simulink model "Q4_V2"  (R2021b)
settings: Solver=VariableStepAuto  StartTime=0.0  StopTime=10  MaxStep=0.0001  RelTol=1e-3
undefined symbols (not defined in the file): a0, a1, a2, b, P0, theta_zero, wn, zeta
libraries: cstblocks x2
settings Model: Creator=mahdi  LastModifiedBy=mahdi

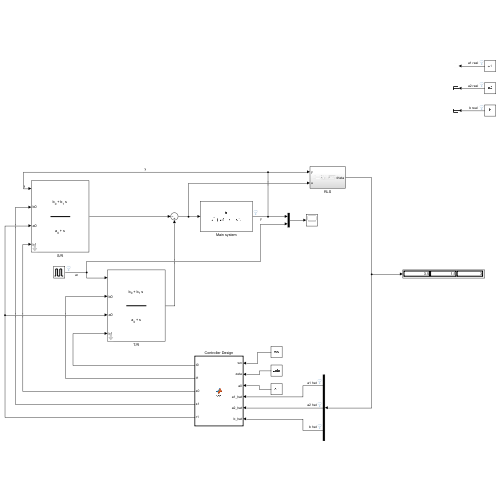
[thumbnail: Simulink's stored preview of the top-level diagram]
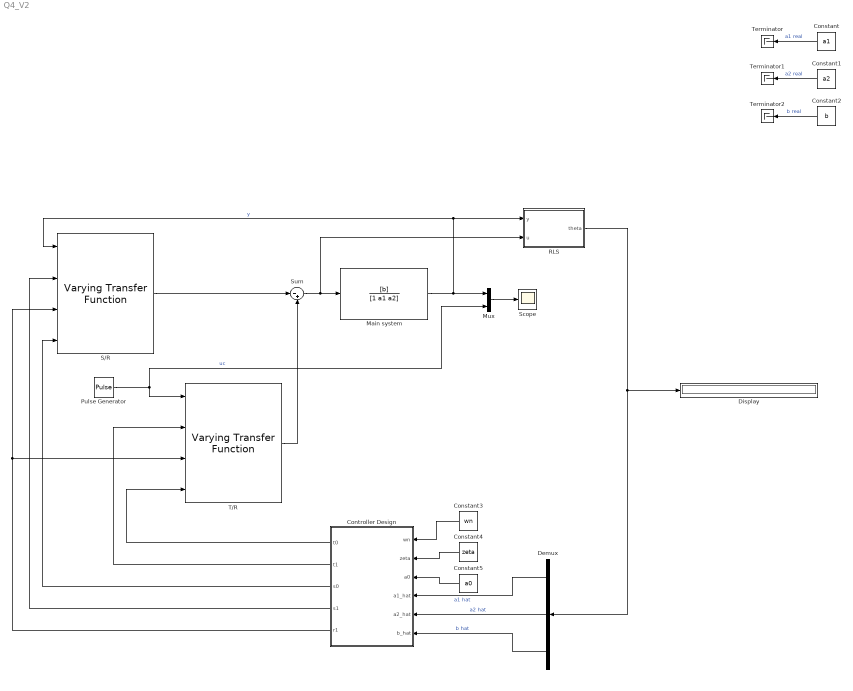
== system Q4_V2 ==
  Constant : Constant  Value=a1
  Constant1 : Constant  Value=a2
  Constant2 : Constant  Value=b
  Constant3 : Constant  Value=wn
  Constant4 : Constant  Value=zeta
  Constant5 : Constant  Value=a0
  Controller Design : MATLAB Function  TreatAsAtomicUnit=on
  Demux : Demux  Outputs=3
  Display : Display
  Main system : TransferFcn  Numerator=[b]  Denominator=[1 a1 a2]
  Mux : Mux  Inputs=2
  Pulse Generator : DiscretePulseGenerator  PulseType=Time based  Period=5  PulseWidth=50
  RLS : Subsystem
  S/R : cstblocks/Linear Parameter Varying/Varying Transfer Function  N=1
  Scope : Scope
  Sum : Sum  Inputs=|-+
  T/R : cstblocks/Linear Parameter Varying/Varying Transfer Function  N=1
  Terminator : Terminator
  Terminator1 : Terminator
  Terminator2 : Terminator
  wires:
  Main system/1 -> RLS/1(y), S/R/1, Mux/1  "y"
  Pulse Generator/1 -> T/R/1, Mux/2  "uc"
  Controller Design/5(r1) -> T/R/3, S/R/3
  Controller Design/3(s0) -> S/R/4
  Controller Design/4(s1) -> S/R/2
  Controller Design/1(t0) -> T/R/4
  Controller Design/2(t1) -> T/R/2
  S/R/1 -> Sum/1
  T/R/1 -> Sum/2
  Sum/1 -> RLS/2(u), Main system/1
  Mux/1 -> Scope/1
  Constant/1 -> Terminator/1  "a1 real"
  Constant1/1 -> Terminator1/1  "a2 real"
  Constant2/1 -> Terminator2/1  "b real"
  Constant5/1 -> Controller Design/3(a0)
  Constant4/1 -> Controller Design/2(zeta)
  Constant3/1 -> Controller Design/1(wn)
  Demux/1 -> Controller Design/4(a1_hat)  "a1 hat"
  Demux/2 -> Controller Design/5(a2_hat)  "a2 hat"
  Demux/3 -> Controller Design/6(b_hat)  "b hat"
  RLS/1(theta) -> Demux/1, Display/1

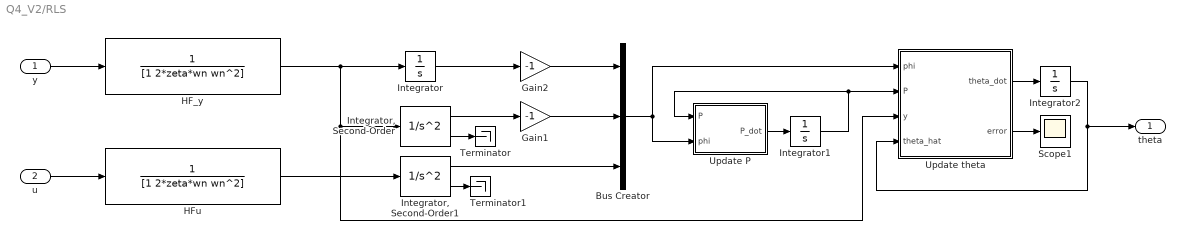
== system Q4_V2/RLS ==
  y : Inport
  u : Inport  Port=2
  Bus Creator : BusCreator  Inputs=3
  Gain1 : Gain  Gain=-1
  Gain2 : Gain  Gain=-1
  HF_y : TransferFcn  Denominator=[1 2*zeta*wn wn^2]
  HFu : TransferFcn  Denominator=[1 2*zeta*wn wn^2]
  Integrator : Integrator
  "Integrator, Second-Order" : SecondOrderIntegrator
  "Integrator, Second-Order1" : SecondOrderIntegrator
  Integrator1 : Integrator  InitialCondition=P0
  Integrator2 : Integrator  InitialCondition=theta_zero
  Scope1 : Scope
  Terminator : Terminator
  Terminator1 : Terminator
  Update P : MATLAB Function  TreatAsAtomicUnit=on
  Update theta : MATLAB Function  TreatAsAtomicUnit=on
  theta : Outport
  wires:
  "Integrator, Second-Order"/1 -> Gain1/1
  Bus Creator/1 -> Update P/2(phi), Update theta/1(phi)
  y/1 -> HF_y/1
  Integrator1/1 -> Update theta/2(P), Update P/1(P)
  Update theta/2(error) -> Scope1/1
  HF_y/1 -> "Integrator, Second-Order"/1, Update theta/3(y), Integrator/1
  "Integrator, Second-Order1"/2 -> Terminator1/1
  "Integrator, Second-Order1"/1 -> Bus Creator/3
  Integrator2/1 -> theta/1, Update theta/4(theta_hat)
  Update P/1(P_dot) -> Integrator1/1
  Update theta/1(theta_dot) -> Integrator2/1
  HFu/1 -> "Integrator, Second-Order1"/1
  Gain1/1 -> Bus Creator/2
  Integrator/1 -> Gain2/1
  Gain2/1 -> Bus Creator/1
  u/1 -> HFu/1
  "Integrator, Second-Order"/2 -> Terminator/1

== matlab function Q4_V2/RLS/Update P ==
  data: P input; phi input; P_dot output
function P_dot = fcn(P,phi)
    alpha = 1;
    P_dot = alpha * P - P * phi * phi.' * P;

== matlab function Q4_V2/Controller Design ==
  data: wn input; zeta input; a0 input; t0 output; t1 output; s0 output; s1 output; a1_hat input; r1 output; a2_hat input; b_hat input
function [t0, t1, s0, s1, r1] = fcn(wn, zeta, a0, a1_hat,a2_hat,b_hat)
%     wn=7.5;
%     zeta=0.7;
%     a0 = 0;
%     am1=2*zeta*wn;
%     am2=wn^2;
%     bm=wn^2;

    r1 = 2 * zeta * wn + a0 - a1_hat;
    s0 = (a0 * 2 * zeta*wn + wn^2 - a1_hat*r1-a2_hat)/b_hat;
    s1 = (wn^2 * a0 -a2_hat*r1)/b_hat;

    t0 = wn^2/b_hat;
    t1 = a0 * wn^2/b_hat;

== matlab function Q4_V2/RLS/Update theta ==
  data: phi input; P input; y input; theta_dot output; theta_hat input; error output
function [theta_dot,error] = fcn(phi, P, y, theta_hat)
    error = y - phi.' * theta_hat;
    theta_dot = P * phi * error;
